simulink model "MI_controle_W_T_I_startup"  (R2015a)
settings: Solver=ode45  StartTime=0.0  StopTime=4.5  RelTol=1e-3
values from neighbouring files (symbols this model uses):
  FLrd_0 = FLr_dq_0    [MI_controle_W_I_T_inicio.m]    (also in MI_controle_W_I_inicio.m; MI_controle_W_I_startup_inicio.m; MI_controle_W_Inicio.m; MI_controle_W_T_I_startup_inicio.m)
  J = 0.025    [MI_controle_W_I_T_inicio.m]    (also in MI_controle_W_I_inicio.m; MI_controle_W_I_startup_inicio.m; MI_controle_W_Inicio.m; MI_controle_W_T_I_startup_inicio.m)
  Ki = (Wc^2*J)/(k*sqrt(1+tan(MF)^2))    [MI_controle_W_I_T_inicio.m]    (also in MI_controle_W_I_inicio.m; MI_controle_W_I_startup_inicio.m; MI_controle_W_Inicio.m; MI_controle_W_T_I_startup_inicio.m)
  Kif = Kii    [MI_controle_W_T_I_startup_inicio.m]
  Kii = Wci*(Wci*sigma*Ls + Rs*tanMF)/sqrt(tanMF^2 + 1)    [MI_controle_W_I_T_inicio.m]    (also in MI_controle_W_I_inicio.m; MI_controle_W_I_startup_inicio.m; MI_controle_W_T_I_startup_inicio.m = Wci*(Wci*sigma*Ls + Rs*tanMFi)/sqrt(tanMFi^2 + 1))
  Kiii = Wcii*(Wcii*sigma*Ls + Rs*tanMF)/sqrt(tanMF^2 + 1)    [MI_controle_W_I_T_inicio.m]    (also in MI_controle_W_T_I_startup_inicio.m = Wcii*(Wcii*sigma*Ls + Rs*tanMFii)/sqrt(tanMFii^2 + 1))
  Kp = Ki*tan(MF)/Wc    [MI_controle_W_I_T_inicio.m]    (also in MI_controle_W_I_inicio.m; MI_controle_W_I_startup_inicio.m; MI_controle_W_Inicio.m; MI_controle_W_T_I_startup_inicio.m)
  Kpf = Kpi    [MI_controle_W_T_I_startup_inicio.m]
  Kpi = (Kii/Wci)*(Wci*sigma*Ls*tanMF - Rs)/(Wci*sigma*Ls + Rs*tanMF)    [MI_controle_W_I_T_inicio.m]    (also in MI_controle_W_I_inicio.m; MI_controle_W_I_startup_inicio.m; MI_controle_W_T_I_startup_inicio.m = (Kii/Wci)*(Wci*sigma*Ls*tanMFi - Rs)/(Wci*sigma*Ls + Rs*tanM)
  Kpii = (Kiii/Wcii)*(Wcii*sigma*Ls*tanMF - Rs)/(Wcii*sigma*Ls + Rs*tanMF)    [MI_controle_W_I_T_inicio.m]    (also in MI_controle_W_T_I_startup_inicio.m = (Kiii/Wcii)*(Wcii*sigma*Ls*tanMFii - Rs)/(Wcii*sigma*Ls + Rs)
  Lm = Xm/Wsyn    (= 0.368708951496)    [MI_controle_W_I_T_inicio.m]    (also in MI_controle_W_I_inicio.m; MI_controle_W_I_startup_inicio.m; MI_controle_W_Inicio.m; MI_controle_W_T_I_startup_inicio.m)
  Lr = (Xlr + Xm)/Wsyn    (= 0.380831252995)    [MI_controle_W_I_T_inicio.m]    (also in MI_controle_W_I_inicio.m; MI_controle_W_I_startup_inicio.m; MI_controle_W_Inicio.m; MI_controle_W_T_I_startup_inicio.m)
  Minv = inv(M)    [MI_controle_W_I_T_inicio.m]    (also in MI_controle_W_I_inicio.m; MI_controle_W_I_startup_inicio.m; MI_controle_W_Inicio.m; MI_controle_W_T_I_startup_inicio.m)
  p = 4    [MI_controle_W_I_T_inicio.m]    (also in MI_controle_W_I_inicio.m; MI_controle_W_I_startup_inicio.m; MI_controle_W_Inicio.m; MI_controle_W_T_I_startup_inicio.m)
  Rs = 1.77    [MI_controle_W_I_T_inicio.m]    (also in MI_controle_W_I_inicio.m; MI_controle_W_I_startup_inicio.m; MI_controle_W_Inicio.m; MI_controle_W_T_I_startup_inicio.m)
  tau_r = Lr/Rr    (= 0.284202427608)    [MI_controle_W_I_T_inicio.m]    (also in MI_controle_W_I_inicio.m; MI_controle_W_I_startup_inicio.m; MI_controle_W_Inicio.m; MI_controle_W_T_I_startup_inicio.m)
  Tem_n = (p/2)*Lm*(Isq_0*Ird_0-Isd_0*Irq_0)    [MI_controle_W_I_startup_inicio.m]    (also in MI_controle_W_T_I_startup_inicio.m)
  Wmech_n = (2/p)*(1-s)*Wsyn    (= 185.253435597)    [MI_controle_W_I_startup_inicio.m]    (also in MI_controle_W_T_I_startup_inicio.m)
settings Model: Creator=range  LastModifiedBy=range

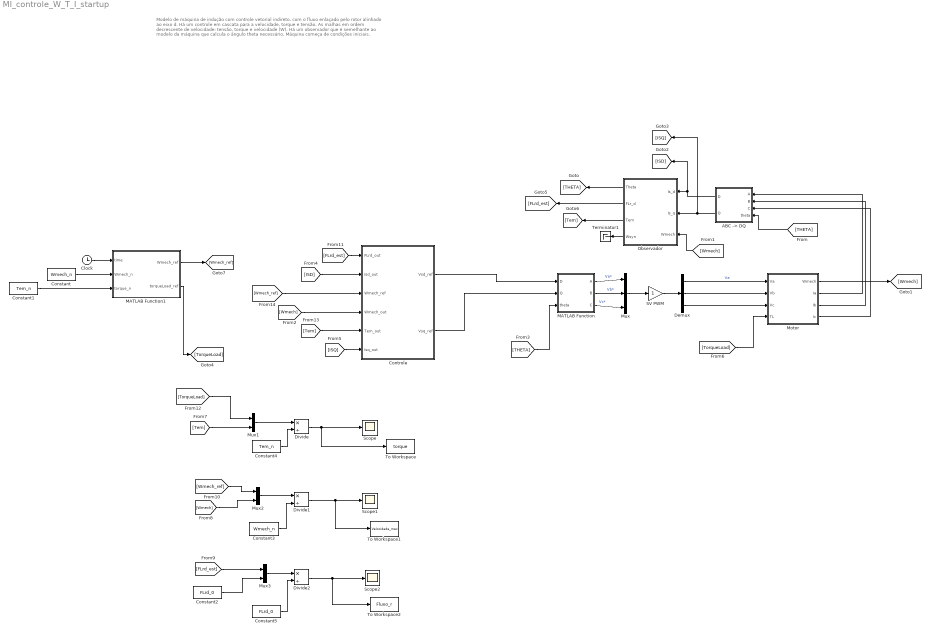
== system MI_controle_W_T_I_startup ==
  note: Modelo de máquina de indução com controle vetorial indireto.
      | com o fluxo enlaçado pelo rotor alinhado
      | ao eixo d.
      | Há um controle em cascata para a velocidade, torque e tensão.
      | As malhas em ordem decrescente de velocidade: tensão, torque e velocidade (W).
      | Há um observador que é semelhante ao modelo da máquina
      | que calcula o ângulo theta necessário.
      | Máquina começa de condições iniciais.
  "ABC -> DQ" : MATLAB Function  TreatAsAtomicUnit=on
  Clock : Clock
  Constant : Constant  Value=Wmech_n
  Constant1 : Constant  Value=Tem_n
  Constant2 : Constant  Value=FLrd_0
  Constant3 : Constant  Value=Wmech_n
  Constant4 : Constant  Value=Tem_n
  Constant5 : Constant  Value=FLrd_0
  Controle : Subsystem
  Demux : Demux  Outputs=3
  Divide : Product  Inputs=*/
  Divide1 : Product  Inputs=*/
  Divide2 : Product  Inputs=*/
  MATLAB Function : MATLAB Function  TreatAsAtomicUnit=on
  MATLAB Function1 : MATLAB Function  TreatAsAtomicUnit=on
  Motor : Subsystem
  Mux : Mux  Inputs=3
  Mux1 : Mux  Inputs=2
  Mux2 : Mux  Inputs=2
  Mux3 : Mux  Inputs=2
  Observador : Subsystem
  SV PWM : Gain
  Scope : Scope
  Scope1 : Scope
      settings: SaveName=ScopeData2
  Scope2 : Scope
      settings: SaveName=ScopeData3
  Terminator1 : Terminator
  To Workspace : ToWorkspace  VariableName=torque  SaveFormat=Timeseries  SampleTime=-1
  To Workspace1 : ToWorkspace  VariableName=Velocidade_mec  SaveFormat=Timeseries  SampleTime=-1
  To Workspace2 : ToWorkspace  VariableName=Fluxo_r  SaveFormat=Timeseries  SampleTime=-1
  wires:
  "ABC -> DQ"/1(D) -> [ISD], Observador/1(Is_d)
  "ABC -> DQ"/2(Q) -> [ISQ], Observador/2(Is_q)
  Observador/4(Wsyn) -> Terminator1/1
  MATLAB Function/1(A) -> Mux/1  "Va*"
  MATLAB Function/2(B) -> Mux/2  "Vb*"
  MATLAB Function/3(C) -> Mux/3  "Vc*"
  Demux/1 -> Motor/1(Va)  "Va"
  Demux/2 -> Motor/2(Vb)
  Demux/3 -> Motor/3(Vc)
  Mux/1 -> SV PWM/1
  SV PWM/1 -> Demux/1
  Observador/1(Theta) -> [THETA]
  [THETA] -> "ABC -> DQ"/4(theta)
  Motor/1(Wmech) -> [Wmech]
  [Wmech] -> Observador/3(Wmech)
  [THETA] -> MATLAB Function/3(theta)
  Observador/3(Tem) -> [Tem]
  Motor/2(Ia) -> "ABC -> DQ"/1(A)
  Motor/3(Ib) -> "ABC -> DQ"/2(B)
  Motor/4(Ic) -> "ABC -> DQ"/3(C)
  [TorqueLoad] -> Motor/4(TL)
  [Tem] -> Mux1/2
  Clock/1 -> MATLAB Function1/1(time)
  Constant/1 -> MATLAB Function1/2(Wmech_n)
  Constant1/1 -> MATLAB Function1/3(torque_n)
  MATLAB Function1/2(torqueLoad_ref) -> [TorqueLoad]
  Observador/2(FLr_d) -> [FLrd_est]
  MATLAB Function1/1(Wmech_ref) -> [Wmech_ref]
  [Wmech_ref] -> Mux2/1
  [Wmech] -> Mux2/2
  [FLrd_est] -> Mux3/1
  Constant2/1 -> Mux3/2
  Mux1/1 -> Divide/1
  Divide/1 -> To Workspace/1, Scope/1
  Divide1/1 -> To Workspace1/1, Scope1/1
  Mux2/1 -> Divide1/1
  Mux3/1 -> Divide2/1
  Divide2/1 -> To Workspace2/1, Scope2/1
  Constant4/1 -> Divide/2
  Constant3/1 -> Divide1/2
  Constant5/1 -> Divide2/2
  [TorqueLoad] -> Mux1/1
  [FLrd_est] -> Controle/1(FLrd_out)
  [ISD] -> Controle/2(Isd_out)
  [Wmech] -> Controle/4(Wmech_out)
  [Tem] -> Controle/5(Tem_out)
  [ISQ] -> Controle/6(Isq_out)
  Controle/1(Vsd_ref) -> MATLAB Function/1(D)
  Controle/2(Vsq_ref) -> MATLAB Function/2(Q)
  [Wmech_ref] -> Controle/3(Wmech_ref)

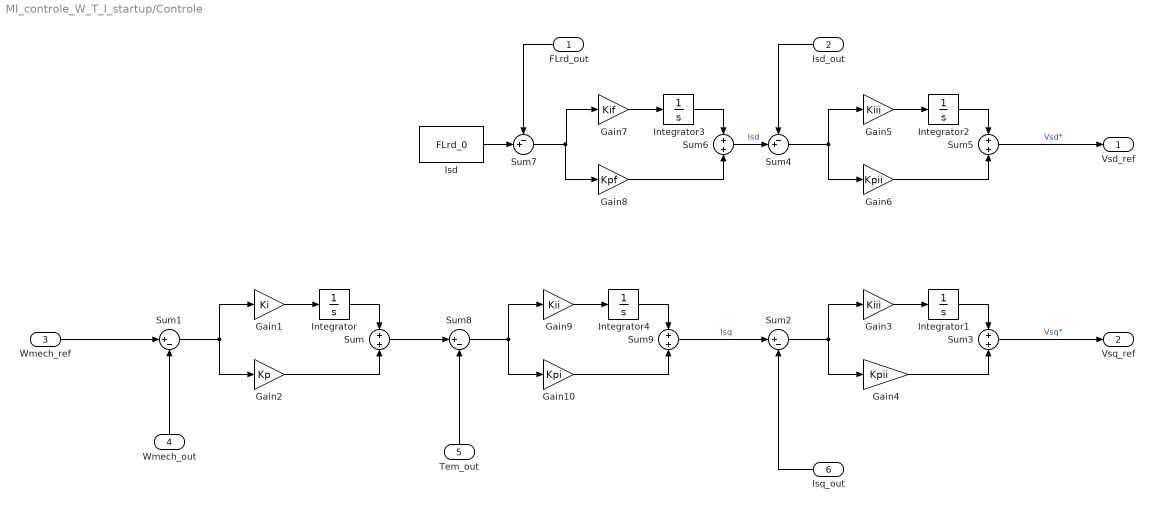
== system MI_controle_W_T_I_startup/Controle ==
  FLrd_out : Inport
  Isd_out : Inport  Port=2
  Wmech_ref : Inport  Port=3
  Wmech_out : Inport  Port=4
  Tem_out : Inport  Port=5
  Isq_out : Inport  Port=6
  Gain1 : Gain  Gain=Ki
  Gain10 : Gain  Gain=Kpi
  Gain2 : Gain  Gain=Kp
  Gain3 : Gain  Gain=Kiii
  Gain4 : Gain  Gain=Kpii
  Gain5 : Gain  Gain=Kiii
  Gain6 : Gain  Gain=Kpii
  Gain7 : Gain  Gain=Kif
  Gain8 : Gain  Gain=Kpf
  Gain9 : Gain  Gain=Kii
  Integrator{,1..4} (5 alike) : Integrator  InitialCondition=0.0
  Isd : Constant  Value=FLrd_0
  Sum{,3,5..6,9} (5 alike) : Sum  Inputs=+|+
  Sum1 : Sum  Inputs=|+-
  Sum2 : Sum  Inputs=|+-
  Sum4 : Sum  Inputs=-+|
  Sum7 : Sum  Inputs=-+|
  Sum8 : Sum  Inputs=|+-
  Vsd_ref : Outport
  Vsq_ref : Outport  Port=2
  wires:
  Sum9/1 -> Sum2/1  "Isq"
  Sum5/1 -> Vsd_ref/1  "Vsd*"
  Isd_out/1 -> Sum4/1
  Gain2/1 -> Sum/2
  Gain4/1 -> Sum3/2
  Sum3/1 -> Vsq_ref/1  "Vsq*"
  Sum4/1 -> Gain5/1, Gain6/1
  Wmech_out/1 -> Sum1/2
  Isq_out/1 -> Sum2/2
  Sum2/1 -> Gain3/1, Gain4/1
  Integrator1/1 -> Sum3/1
  Integrator/1 -> Sum/1
  Sum1/1 -> Gain1/1, Gain2/1
  Gain3/1 -> Integrator1/1
  Gain5/1 -> Integrator2/1
  Integrator2/1 -> Sum5/1
  Gain6/1 -> Sum5/2
  Gain1/1 -> Integrator/1
  Isd/1 -> Sum7/2
  FLrd_out/1 -> Sum7/1
  Gain7/1 -> Integrator3/1
  Gain8/1 -> Sum6/2
  Sum7/1 -> Gain8/1, Gain7/1
  Sum6/1 -> Sum4/2  "Isd"
  Integrator3/1 -> Sum6/1
  Integrator4/1 -> Sum9/1
  Gain10/1 -> Sum9/2
  Sum/1 -> Sum8/1
  Tem_out/1 -> Sum8/2
  Sum8/1 -> Gain9/1, Gain10/1
  Gain9/1 -> Integrator4/1
  Wmech_ref/1 -> Sum1/1

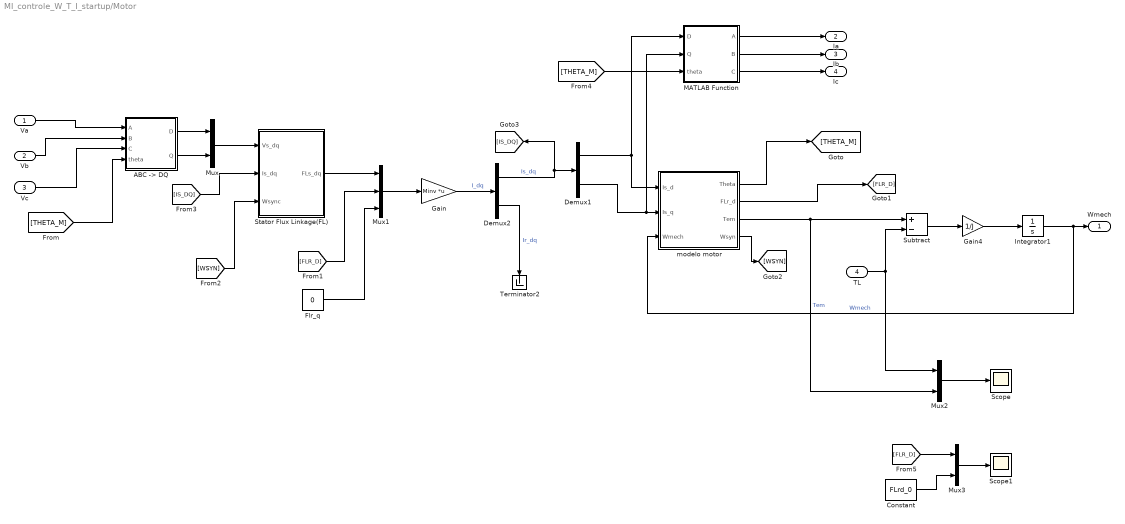
== system MI_controle_W_T_I_startup/Motor ==
  Va : Inport
  Vb : Inport  Port=2
  Vc : Inport  Port=3
  TL : Inport  Port=4
  "ABC -> DQ" : MATLAB Function  TreatAsAtomicUnit=on
  Constant : Constant  Value=FLrd_0
  Demux1 : Demux  Outputs=2
  Demux2 : Demux  Outputs=2
  Flr_q : Constant  Value=0
  Gain : Gain  Gain=Minv  Multiplication=Matrix(K*u)
  Gain4 : Gain  Gain=1/J
  Integrator1 : Integrator  InitialCondition=0.0
  MATLAB Function : MATLAB Function  TreatAsAtomicUnit=on
  Mux : Mux  Inputs=2
  Mux1 : Mux  Inputs=3
  Mux2 : Mux  Inputs=2
  Mux3 : Mux  Inputs=2
  Scope : Scope
  Scope1 : Scope
      settings: SaveName=ScopeData4
  "Stator Flux Linkage(FL) " : Subsystem
  Subtract : Sum  Inputs=+-
  Terminator2 : Terminator
  modelo motor : Subsystem
  Wmech : Outport
  Ia : Outport  Port=2
  Ib : Outport  Port=3
  Ic : Outport  Port=4
  wires:
  Va/1 -> "ABC -> DQ"/1(A)
  Vb/1 -> "ABC -> DQ"/2(B)
  Vc/1 -> "ABC -> DQ"/3(C)
  modelo motor/2(FLr_d) -> [FLR_D]
  Mux2/1 -> Scope/1
  modelo motor/3(Tem) -> Subtract/1, Mux2/2  "Tem"
  Subtract/1 -> Gain4/1
  Gain4/1 -> Integrator1/1
  Integrator1/1 -> modelo motor/3(Wmech), Wmech/1  "Wmech"
  modelo motor/1(Theta) -> [THETA_M]
  [THETA_M] -> "ABC -> DQ"/4(theta)
  "ABC -> DQ"/1(D) -> Mux/1
  "ABC -> DQ"/2(Q) -> Mux/2
  Mux/1 -> "Stator Flux Linkage(FL) "/1(Vs_dq)
  Gain/1 -> Demux2/1  "I_dq"
  "Stator Flux Linkage(FL) "/1(FLs_dq) -> Mux1/1
  Demux2/2 -> Terminator2/1  "Ir_dq"
  Mux1/1 -> Gain/1
  [FLR_D] -> Mux1/2
  modelo motor/4(Wsyn) -> [WSYN]
  [WSYN] -> "Stator Flux Linkage(FL) "/3(Wsync)
  Flr_q/1 -> Mux1/3
  Demux2/1 -> [IS_DQ], Demux1/1  "Is_dq"
  Demux1/1 -> MATLAB Function/1(D), modelo motor/1(Is_d)
  Demux1/2 -> MATLAB Function/2(Q), modelo motor/2(Is_q)
  [IS_DQ] -> "Stator Flux Linkage(FL) "/2(Is_dq)
  [THETA_M] -> MATLAB Function/3(theta)
  MATLAB Function/1(A) -> Ia/1
  MATLAB Function/3(C) -> Ic/1
  MATLAB Function/2(B) -> Ib/1
  TL/1 -> Mux2/1, Subtract/2
  Mux3/1 -> Scope1/1
  [FLR_D] -> Mux3/1
  Constant/1 -> Mux3/2

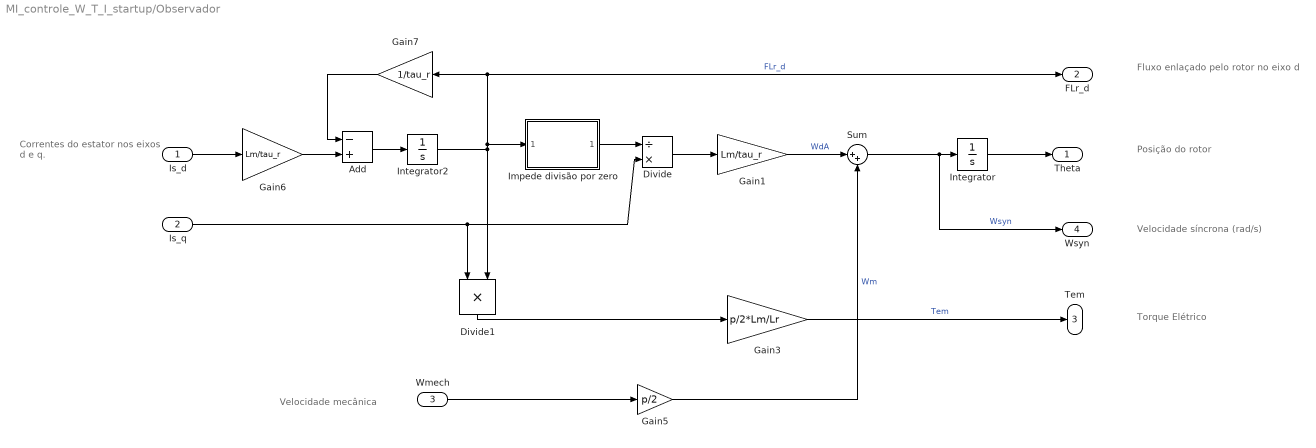
== system MI_controle_W_T_I_startup/Observador ==
  note: Correntes do estator
      | nos eixos d e q.
  note: Velocidade mecânica
  note: Torque Elétrico
  note: Velocidade síncrona (rad/s)
  note: Posição do rotor
  note: Fluxo enlaçado pelo rotor no eixo d
  Is_d : Inport
  Is_q : Inport  Port=2
  Wmech : Inport  Port=3
  Add : Sum  Inputs=-+
  Divide : Product  Inputs=/*
  Divide1 : Product  Inputs=**
  Gain1 : Gain  Gain=Lm/tau_r
  Gain3 : Gain  Gain=p/2*Lm/Lr
  Gain5 : Gain  Gain=p/2
  Gain6 : Gain  Gain=Lm/tau_r
  Gain7 : Gain  Gain=1/tau_r
  Impede divisão por zero : MATLAB Function  TreatAsAtomicUnit=on
  Integrator : Integrator
  Integrator2 : Integrator
  Sum : Sum  Inputs=|++
  Theta : Outport
  FLr_d : Outport  Port=2
  Tem : Outport  Port=3
  Wsyn : Outport  Port=4
  wires:
  Is_q/1 -> Divide/2, Divide1/1
  Integrator/1 -> Theta/1
  Sum/1 -> Wsyn/1, Integrator/1  "Wsyn"
  Add/1 -> Integrator2/1
  Gain1/1 -> Sum/1  "WdA"
  Is_d/1 -> Gain6/1
  Gain7/1 -> Add/1
  Gain6/1 -> Add/2
  Integrator2/1 -> FLr_d/1, Gain7/1, Impede divisão por zero/1(FLrd_in), Divide1/2  "FLr_d"
  Divide1/1 -> Gain3/1
  Gain3/1 -> Tem/1  "Tem"
  Divide/1 -> Gain1/1
  Wmech/1 -> Gain5/1
  Gain5/1 -> Sum/2  "Wm"
  Impede divisão por zero/1(FLrd_out) -> Divide/1

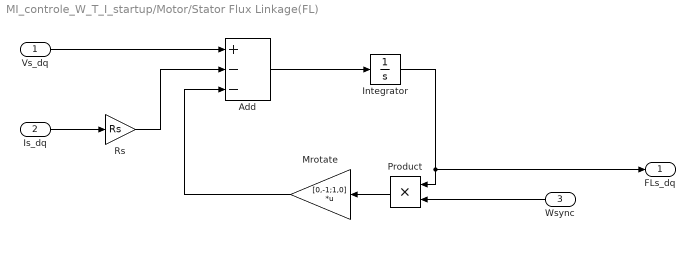
== system MI_controle_W_T_I_startup/Motor/Stator Flux Linkage(FL)  ==
  Vs_dq : Inport
  Is_dq : Inport  Port=2
  Wsync : Inport  Port=3
  Add : Sum  Inputs=+--
  Integrator : Integrator  InitialCondition=[0;0]
  Mrotate : Gain  Gain=[0,-1;1,0]  Multiplication=Matrix(K*u)
  Product : Product
  Rs : Gain  Gain=Rs
  FLs_dq : Outport
  wires:
  Vs_dq/1 -> Add/1
  Product/1 -> Mrotate/1
  Rs/1 -> Add/2
  Add/1 -> Integrator/1
  Mrotate/1 -> Add/3
  Integrator/1 -> FLs_dq/1, Product/1
  Wsync/1 -> Product/2
  Is_dq/1 -> Rs/1

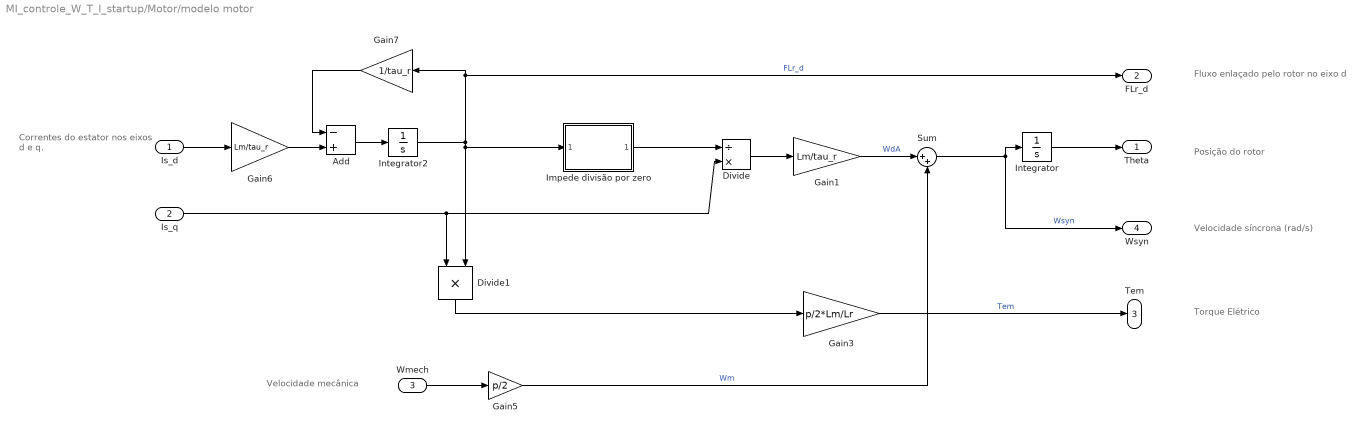
== system MI_controle_W_T_I_startup/Motor/modelo motor ==
  note: Correntes do estator
      | nos eixos d e q.
  note: Velocidade mecânica
  note: Torque Elétrico
  note: Velocidade síncrona (rad/s)
  note: Posição do rotor
  note: Fluxo enlaçado pelo rotor no eixo d
  Is_d : Inport
  Is_q : Inport  Port=2
  Wmech : Inport  Port=3
  Add : Sum  Inputs=-+
  Divide : Product  Inputs=/*
  Divide1 : Product  Inputs=**
  Gain1 : Gain  Gain=Lm/tau_r
  Gain3 : Gain  Gain=p/2*Lm/Lr
  Gain5 : Gain  Gain=p/2
  Gain6 : Gain  Gain=Lm/tau_r
  Gain7 : Gain  Gain=1/tau_r
  Impede divisão por zero : MATLAB Function  TreatAsAtomicUnit=on
  Integrator : Integrator
  Integrator2 : Integrator
  Sum : Sum  Inputs=|++
  Theta : Outport
  FLr_d : Outport  Port=2
  Tem : Outport  Port=3
  Wsyn : Outport  Port=4
  wires:
  Is_q/1 -> Divide/2, Divide1/1
  Integrator/1 -> Theta/1
  Sum/1 -> Wsyn/1, Integrator/1  "Wsyn"
  Add/1 -> Integrator2/1
  Gain1/1 -> Sum/1  "WdA"
  Is_d/1 -> Gain6/1
  Gain7/1 -> Add/1
  Gain6/1 -> Add/2
  Integrator2/1 -> Divide1/2, Impede divisão por zero/1(FLrd_in), Gain7/1, FLr_d/1  "FLr_d"
  Divide1/1 -> Gain3/1
  Gain3/1 -> Tem/1  "Tem"
  Divide/1 -> Gain1/1
  Wmech/1 -> Gain5/1
  Gain5/1 -> Sum/2  "Wm"
  Impede divisão por zero/1(FLrd_out) -> Divide/1

== matlab function MI_controle_W_T_I_startup/ABC -> DQ ==
  data: A input; D output; B input; C input; theta input; Q output
function [D,Q] = ABCtoDQ(A,B,C,theta)
%Transformação de grandezas trifásicas para os eixos D e Q.

DQ = sqrt(2/3)*[cos(theta), cos(theta-2*pi/3), cos(theta-4*pi/3);...
               -sin(theta),-sin(theta-2*pi/3),-sin(theta-4*pi/3)]*[A;B;C];
D = DQ(1);
Q = DQ(2);

== matlab function MI_controle_W_T_I_startup/Motor/ABC -> DQ ==
  data: A input; D output; B input; C input; theta input; Q output
function [D,Q] = ABCtoDQ(A,B,C,theta)
%Transformação de grandezas trifásicas para os eixos D e Q.

DQ = sqrt(2/3)*[cos(theta), cos(theta-2*pi/3), cos(theta-4*pi/3);...
               -sin(theta),-sin(theta-2*pi/3),-sin(theta-4*pi/3)]*[A;B;C];
D = DQ(1);
Q = DQ(2);

== matlab function MI_controle_W_T_I_startup/MATLAB Function ==
  data: D input; A output; Q input; theta input; B output; C output
function [A,B,C] = DQtoABC(D,Q,theta)
%Transformação inversa de Park.

ABC = sqrt(2/3)*[cos(theta),          -sin(theta); ...
                 cos(theta + 4*pi/3), -sin(theta + 4*pi/3); ...
                 cos(theta + 2*pi/3), -sin(theta + 2*pi/3)]*[D;Q];
A = ABC(1);
B = ABC(2);
C = ABC(3);

== matlab function MI_controle_W_T_I_startup/Motor/MATLAB Function ==
  data: D input; A output; Q input; theta input; B output; C output
function [A,B,C] = DQtoABC(D,Q,theta)
%Transformação inversa de Park.

ABC = sqrt(2/3)*[cos(theta),          -sin(theta); ...
                 cos(theta + 4*pi/3), -sin(theta + 4*pi/3); ...
                 cos(theta + 2*pi/3), -sin(theta + 2*pi/3)]*[D;Q];
A = ABC(1);
B = ABC(2);
C = ABC(3);

== matlab function MI_controle_W_T_I_startup/Motor/modelo motor/Impede divisão por zero ==
  data: FLrd_in input; FLrd_out output
function FLrd_out = iszero(FLrd_in)
%Detecta se fluxo enlaçado pelo rotor é zero e impede a divisão por zero.
if FLrd_in == 0.0
    FLrd_out = 1.0;
else
    FLrd_out = FLrd_in;
end

== matlab function MI_controle_W_T_I_startup/MATLAB Function1 ==
  data: time input; Wmech_ref output; torqueLoad_ref output; Wmech_n input; torque_n input
function [Wmech_ref, torqueLoad_ref]= geradorderef(time, Wmech_n, torque_n)
% Gerador de referências para torque da carga e velocidade mecânica.

if (time >= 1.5) && (time < 2.5)
    Wmech_ref = Wmech_n/4;
    torqueLoad_ref = 0.0;
elseif (time >= 2.5) && (time < 3.5)
    Wmech_ref = Wmech_n/2;
    torqueLoad_ref = 0.0;
elseif time >= 3.5
    Wmech_ref = Wmech_n/2;
    torqueLoad_ref = torque_n/4;
else
    Wmech_ref = 0.0;
    torqueLoad_ref = 0.0;
end
   
end

== matlab function MI_controle_W_T_I_startup/Observador/Impede divisão por zero ==
  data: FLrd_in input; FLrd_out output
function FLrd_out = iszero(FLrd_in)
%Detecta se fluxo enlaçado pelo rotor é zero e impede a divisão por zero.
if FLrd_in == 0.0
    FLrd_out = 1.0;
else
    FLrd_out = FLrd_in;
end
